simulink model "sampleModel364"  (R2021b)
settings: Solver=VariableStepAuto  StartTime=0.0  StopTime=10.0  RelTol=1e-3
undefined symbols (not defined in the file or in its folder): DiscIntNeverNeededParam, Newton, Raphson
libraries: simulink x11, slpidlib x2
settings Model: Creator=user  LastModifiedBy=user

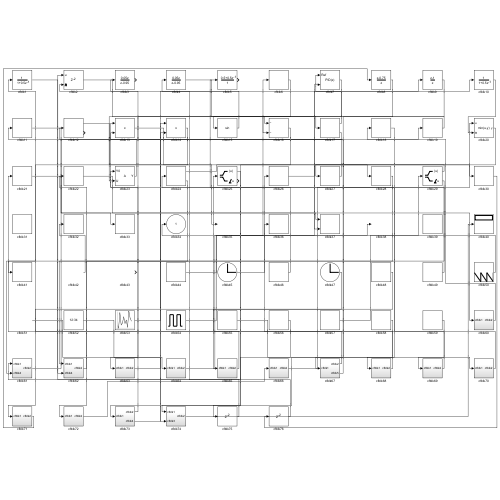
[thumbnail: Simulink's stored preview of the top-level diagram]
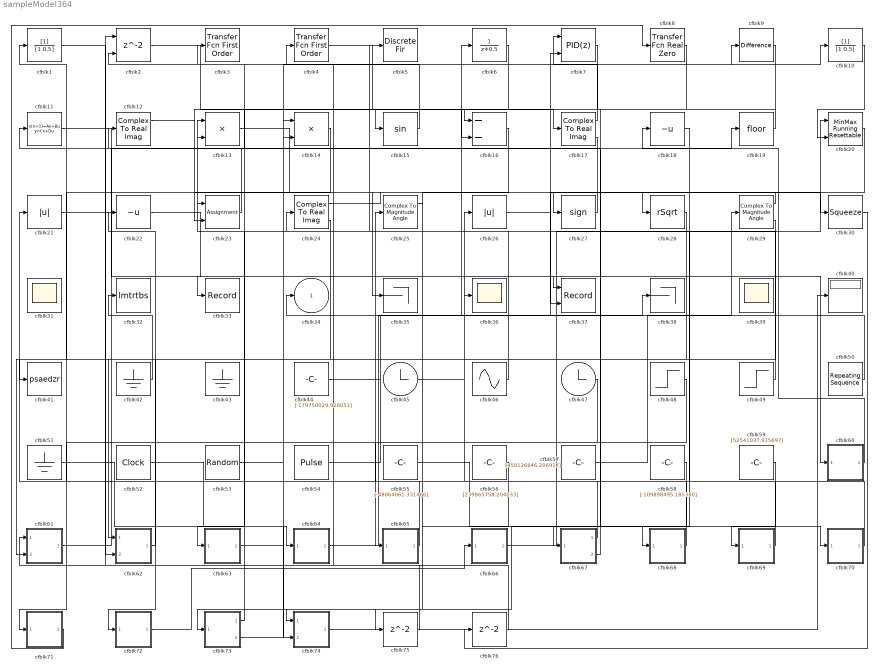
== system sampleModel364 ==
  cfblk1 : DiscreteFilter  SampleTime=1
  cfblk10 : DiscreteFilter  SampleTime=1
  cfblk11 : DiscreteStateSpace
  cfblk12 : ComplexToRealImag
  cfblk13 : Product
  cfblk14 : Product
  cfblk15 : Trigonometry
  cfblk16 : Sum  Inputs=--
  cfblk17 : ComplexToRealImag
  cfblk18 : UnaryMinus
  cfblk19 : Rounding
  cfblk2 : Delay  ShowEnablePort=on  SampleTime=1
      settings: InputPortMap=u0,e6
  cfblk20 : simulink/Math Operations/MinMax Running Resettable  Function=min  vinit=0.0
  cfblk21 : Abs
  cfblk22 : UnaryMinus
  cfblk23 : Assignment  DiagnosticForDimensions=Warning  IndexOptions=Index vector (dialog)  Indices=1  OutputSizes=1
  cfblk24 : ComplexToRealImag
  cfblk25 : ComplexToMagnitudeAngle
  cfblk26 : Abs
  cfblk27 : Signum
  cfblk28 : Sqrt  Operator=rSqrt  AlgorithmType=Newton-Raphson  SaturateOnIntegerOverflow=on
  cfblk29 : ComplexToMagnitudeAngle
  cfblk3 : simulink/Discrete/Transfer Fcn First Order  PoleZ=0.95  ICPrevOutput=0.0  DoSatur=off
  cfblk30 : Squeeze
  cfblk31 : Scope
      settings: Floating=on
  cfblk32 : ToWorkspace  VariableName=lmtrtbs  SaveFormat=Timeseries  SampleTime=-1
  cfblk33 : Record  FileSettingsInternal="{\"entries\":[{\"content\":{\"excelSettings\":{\"content\":{},\"type\":\"Streamout.ExcelSettings\"}},\"type\":\"Streamout.FileSettingStorage\",\"uuid\":\"efb9514b-eb39-49fb-8193-be4ff1269e7a\"}],\"packageUris\":[\"http://schema.mathworks.com/mf0/streamout_blocks/R2020a\"],\"version\":\"1.0\"}"  SignalsInternal="{\"entries\":[{\"content\":{\"signals\":[{\"content\":{\"blockPath\":[\"sampleModel364/cfblk33\"],\"channel\":[],\"dimensions\":[1],\"domain\":\"sampleModel364/cfblk33\",\"lineColor\":\"#0072bd\",\"plots\":[1],\"port\":1,\"sid\":[\"\"],\"signalID\":15049,\"signalName\":\"cfblk21\"},\"type\":\"RecordBlkView.Signal\",\"uuid\":\"19dc1517-5a93-4edc-820c-dcf5ac46ff94\"}]},\"type\":\"RecordBlkView.InputSignals\",\"uuid\":\"c811df6d-3595-4dee-9df3-0c2b135d4dd7\"}],\"packageUris\":[\"http://schema.mathworks.com/mf0/streamout_blocks/R2020a\"],\"version\":\"1.0\"}"  VisualizationBindings="{\"sparklinesplugin\":{\"info\":[{\"bindingParametersList\":[],\"subplotID\":1}]}}"
  cfblk35 : Terminator
  cfblk36 : Scope
  cfblk37 : Record  FileSettingsInternal="{\"entries\":[{\"content\":{\"excelSettings\":{\"content\":{},\"type\":\"Streamout.ExcelSettings\"}},\"type\":\"Streamout.FileSettingStorage\",\"uuid\":\"e2a7b882-2422-4f38-8975-ecb5b9b0d6a4\"}],\"packageUris\":[\"http://schema.mathworks.com/mf0/streamout_blocks/R2020a\"],\"version\":\"1.0\"}"  Layout=[1 1]  SignalsInternal="{\"entries\":[{\"content\":{\"signals\":[{\"content\":{\"blockPath\":[\"sampleModel364/cfblk37\"],\"channel\":[],\"dimensions\":[1],\"domain\":\"sampleModel364/cfblk37\",\"lineColor\":\"#a2142f\",\"plots\":[1],\"port\":1,\"sid\":[\"\"],\"signalID\":15041,\"signalName\":\"cfblk11\"},\"type\":\"RecordBlkView.Signal\",\"uuid\":\"8bbf27e7-d6ab-404e-982e-e11606491116\"},{\"content\":{\"blockPath\":[\"sampleModel364/cfblk37\"],\"channel\":[],\"dimensions\":[1],\"domain\":\"sampleModel364/cfblk37\",\"lineColor\":\"#139fff\",\"plots\":[1],\"port\":2,\"sid\":[\"\"],\"signalID\":15045,\"signalName\":\"cfblk20\"},\"type\":\"RecordBlkView.Signal\",\"uuid\":\"d022dd17-1fd8-4305-9f89-9d03c1f5384f\"}]},\"type\":\"RecordBlkView.InputSignals\",\"uuid\":\"b0c6aa1a-cfa3-4be9-9be2-43c7654ec479\"}],\"packageUris\":[\"http://schema.mathworks.com/mf0/streamout_blocks/R2020a\"],\"version\":\"1.0\"}"  VisualizationBindings="{\"xyplotplugin\":{\"info\":[{\"series\":[{\"bindingParametersList\":[{\"parameter\":\"X-Axis\",\"signalID\":15041,\"signalName\":\"cfblk11\"},{\"parameter\":\"Y-Axis\",\"signalID\":15045,\"signalName\":\"cfblk20\"}],\"seriesID\":3754}],\"subplotID\":1}]}}"  CompatibilityTag=XY
  cfblk38 : Terminator
  cfblk39 : Scope
      settings: Floating=on
  cfblk4 : simulink/Discrete/Transfer Fcn First Order  PoleZ=0.95  ICPrevOutput=0.0  DoSatur=off
  cfblk40 : Display
  cfblk41 : ToWorkspace  VariableName=psaedzr  SaveFormat=Timeseries  SampleTime=-1
  cfblk42 : Ground
  cfblk43 : Ground
  cfblk44 : Constant  Value=[-179750029.926051]  SampleTime=1
  cfblk45 : Clock
  cfblk46 : Sin  Amplitude=[258865866.152019]  Bias=[76546050.477614]  SampleTime=0
  cfblk47 : Clock
  cfblk48 : Step  Time=[28.000000]  Before=[914174276.713515]  After=[433065925.767623]  SampleTime=0
  cfblk49 : Step  Time=[16.000000]  Before=[-678100885.118563]  After=[625681601.472301]  SampleTime=0
  cfblk5 : DiscreteFir  SampleTime=1
  cfblk50 : simulink/Sources/Repeating Sequence  rep_seq_t=[0 2]  rep_seq_y=[-313407330.897961, -602777563.387411]
  cfblk51 : Ground
  cfblk52 : DigitalClock
  cfblk53 : UniformRandomNumber  Minimum=[-9430328336.158092]  Maximum=[6561492100.222932]  Seed=[48463456.000000]  SampleTime=0.1
  cfblk54 : DiscretePulseGenerator  PulseType=Time based  Amplitude=[255418173.633285]  Period=[59331713.081487]  PulseWidth=5  PhaseDelay=[5.000000]
  cfblk55 : Constant  Value=[-48864061.331466]  SampleTime=1
  cfblk56 : Constant  Value=[239865758.204033]  SampleTime=1
  cfblk57 : Constant  Value=[450126646.206917]  SampleTime=1
  cfblk58 : Constant  Value=[-109898495.185380]  SampleTime=1
  cfblk59 : Constant  Value=[52541037.915697]  SampleTime=1
  cfblk6 : DiscreteTransferFcn  SampleTime=1
  cfblk60 : Subsystem
  cfblk61 : Subsystem
  cfblk62 : Subsystem
  cfblk63 : Subsystem
  cfblk64 : Subsystem
  cfblk65 : Subsystem
  cfblk66 : Subsystem
  cfblk67 : Subsystem
  cfblk68 : Subsystem
  cfblk69 : Subsystem
  cfblk7 : slpidlib/PID Controller (2DOF)  Controller=PID  Form=Parallel  TimeDomain=Discrete-time  UseExternalTs=off  SampleTime=1  IntegratorMethod=Forward Euler  FilterMethod=Forward Euler  ControllerParametersSource=internal  P=1  I=1  D=0  UseFilter=on  N=100  b=1  c=1  TunerSelectOption=Transfer Function Based (PID Tuner App)  InitialConditionSource=internal  InitialConditionForIntegrator=0  InitialConditionForFilter=0  DifferentiatorICPrevScaledInput=0  ExternalReset=none  TrackingMode=off  Kt=1  LimitOutput=off  SatLimitsSource=internal  UpperSaturationLimit=inf  LowerSaturationLimit=-inf  LinearizeAsGain=off  AntiWindupMode=none  Kb=1  POutMin=[]  POutMax=[]  IOutMin=[]  IOutMax=[]  DOutMin=[]  DOutMax=[]  NOutMin=[]  NOutMax=[]  bOutMin=[]  bOutMax=[]  cOutMin=[]  cOutMax=[]  SumOutMin=[]  SumOutMax=[]  SaturationOutMin=[]  SaturationOutMax=[]  PParamMin=[]  PParamMax=[]  IParamMin=[]  IParamMax=[]  DParamMin=[]  DParamMax=[]  NParamMin=[]  NParamMax=[]  bParamMin=[]  bParamMax=[]  cParamMin=[]  cParamMax=[]  KbParamMin=[]  KbParamMax=[]  KtParamMin=[]  KtParamMax=[]  KbOutMin=[]  KbOutMax=[]  KtOutMin=[]  KtOutMax=[]  IntegratorOutMin=[]  IntegratorOutMax=[]  FilterOutMin=[]  FilterOutMax=[]  SumI1OutMin=[]  SumI1OutMax=[]  SumI2OutMin=[]  SumI2OutMax=[]  SumI3OutMin=[]  SumI3OutMax=[]  SumI4OutMin=[]  SumI4OutMax=[]  SumDOutMin=[]  SumDOutMax=[]  Sum1OutMin=[]  Sum1OutMax=[]  Sum2OutMin=[]  Sum2OutMax=[]  Sum3OutMin=[]  Sum3OutMax=[]  DifferentiatorOutMin=[]  DifferentiatorOutMax=[]  FilterDiffOutCoefMin=[]  FilterDiffOutCoefMax=[]  ReciprocalOutMin=[]  ReciprocalOutMax=[]  SumDenOutMin=[]  SumDenOutMax=[]  SumNumOutMin=[]  SumNumOutMax=[]  DivideOutMin=[]  DivideOutMax=[]  UdiffTsProdOutMin=[]  UdiffTsProdOutMax=[]  NTsProdOutMin=[]  NTsProdOutMax=[]  UintegralTsProdOutMin=[]  UintegralTsProdOutMax=[]  UngainTsProdOutMin=[]  UngainTsProdOutMax=[]  IntegratorContinuousStateAttributes=''  IntegratorStateMustResolveToSignalObject=off  IntegratorRTWStateStorageClass=Auto  FilterContinuousStateAttributes=''  FilterStateMustResolveToSignalObject=off  FilterRTWStateStorageClass=Auto  ParallelPVariant=InternalParameters  IdealPVariant=Disabled  IVariant=InternalParameters  DVariant=InternalParameters  bVariant=InternalParameters  cVariant=InternalParameters  IntegratorVariant=Discrete  SatVariant=Disabled  AWVariant=Passthrough  PCopyVariant=Disabled  TRVariant=Disabled  FdbkBlocksVariant=Forward  IdealPFdbkVariant=Disabled  SatFdbkVariant=Disabled  DerivativeFilterVariant=ForwardEulerFilter  NVariant=InternalParameters  NCopyVariant=Disabled  FilterICVariant=InternalICsFilter  IntegratorICVariant=InternalICs  ExternalResetVariant=Disabled  TRSumVariant=Passthrough  SumFdbkVariant=Disabled  SumVariant=Sum_PID  TsampFilterVariant=InternalTs  TsampNgainVariant=Passthrough  TsampIntegralVariant=Passthrough  ExternalSaturationOutDataTypeStr=Inherit: Same as second input
      settings: SourceProductBaseCode=SL
  cfblk70 : Subsystem
  cfblk71 : Subsystem
  cfblk72 : Subsystem
  cfblk73 : Subsystem
  cfblk74 : Subsystem
  cfblk75 : Delay  SampleTime=1
  cfblk76 : Delay  SampleTime=1
  cfblk8 : simulink/Discrete/Transfer Fcn Real Zero  ZeroZ=0.75  ICPrevInput=0.0  DoSatur=off
      settings: SourceProductBaseCode=SL
  cfblk9 : simulink/Discrete/Difference  ICPrevInput=0.0  OutMin=[]  OutMax=[]  OutDataTypeStr=Inherit: Inherit via back propagation  OutDataType=fixdt(1, 16)  OutScaling=2^-10  DoSatur=off
  cfblk34 : Outport
  wires:
  cfblk29/1 -> cfblk27/1
  cfblk64/1(cfblk2) -> cfblk38/1
  cfblk19/1 -> cfblk15/1
  cfblk60/1(cfblk2) -> cfblk18/1
  cfblk56/1 -> cfblk61/1(cfblk1)
  cfblk69/1(cfblk2) -> cfblk5/1
  cfblk58/1 -> cfblk73/1(cfblk1)
  cfblk28/1 -> cfblk61/2(cfblk4)
  cfblk65/1(cfblk2) -> cfblk21/1
  cfblk61/1(cfblk2) -> cfblk19/1
  cfblk49/1 -> cfblk13/1
  cfblk55/1 -> cfblk70/1(cfblk1)
  cfblk66/1(cfblk2) -> cfblk20/1
  cfblk47/1 -> cfblk71/1(cfblk1)
  cfblk45/1 -> cfblk26/1
  cfblk11/1 -> cfblk37/1
  cfblk53/1 -> cfblk14/1
  cfblk51/1 -> cfblk64/1(cfblk1)
  cfblk71/1(cfblk2) -> cfblk8/1
  cfblk20/1 -> cfblk37/2
  cfblk21/1 -> cfblk33/1
  cfblk29/2 -> cfblk62/1(cfblk1)
  cfblk17/1 -> cfblk7/1
  cfblk1/1 -> cfblk62/2(cfblk4)
  cfblk22/1 -> cfblk60/1(cfblk1)
  cfblk72/1(cfblk2) -> cfblk66/1(cfblk1)
  cfblk67/1(cfblk2) -> cfblk1/1
  cfblk42/1 -> cfblk32/1
  cfblk59/1 -> cfblk69/1(cfblk1)
  cfblk70/1(cfblk2) -> cfblk36/1
  cfblk50/1 -> cfblk34/1
  cfblk14/1 -> cfblk41/1
  cfblk68/1(cfblk2) -> cfblk25/1
  cfblk44/1 -> cfblk6/1
  cfblk24/1 -> cfblk30/1
  cfblk73/1(cfblk2) -> cfblk23/1
  cfblk25/1 -> cfblk74/1(cfblk1)
  cfblk62/1(cfblk2) -> cfblk22/1
  cfblk6/1 -> cfblk23/2
  cfblk2/1 -> cfblk16/1
  cfblk48/1 -> cfblk65/1(cfblk1)
  cfblk4/1 -> cfblk17/1
  cfblk10/1 -> cfblk20/2
  cfblk54/1 -> cfblk7/2
  cfblk26/1 -> cfblk9/1
  cfblk74/1(cfblk2) -> cfblk40/1
  cfblk9/1 -> cfblk67/1(cfblk1)
  cfblk18/1 -> cfblk68/1(cfblk1)
  cfblk17/2 -> cfblk11/1
  cfblk67/2(cfblk5) -> cfblk13/2
  cfblk13/1 -> cfblk35/1
  cfblk15/1 -> cfblk2/2
  cfblk24/2 -> cfblk72/1(cfblk1)
  cfblk12/1 -> cfblk28/1
  cfblk63/1(cfblk2) -> cfblk10/1
  cfblk23/1 -> cfblk12/1
  cfblk57/1 -> cfblk29/1
  cfblk27/1 -> cfblk3/1
  cfblk52/1 -> cfblk74/2(cfblk3)
  cfblk73/2(cfblk4) -> cfblk14/2
  cfblk8/1 -> cfblk16/2
  cfblk46/1 -> cfblk4/1
  cfblk7/1 -> cfblk63/1(cfblk1)
  cfblk16/1 -> cfblk75/1
  cfblk75/1 -> cfblk2/1
  cfblk30/1 -> cfblk76/1
  cfblk76/1 -> cfblk24/1

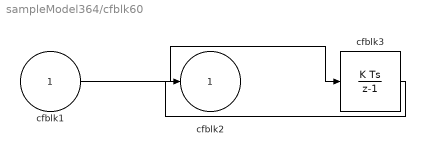
== system sampleModel364/cfblk60 ==
  cfblk1 : Inport
  cfblk3 : DiscreteIntegrator  ICPrevOutput=DiscIntNeverNeededParam  ICPrevScaledInput=DiscIntNeverNeededParam
  cfblk2 : Outport
  wires:
  cfblk1/1 -> cfblk3/1
  cfblk3/1 -> cfblk2/1

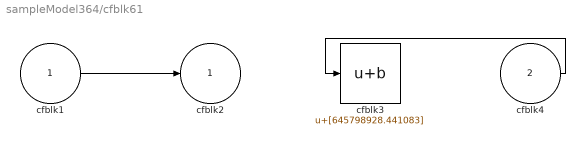
== system sampleModel364/cfblk61 ==
  cfblk1 : Inport
  cfblk4 : Inport  Port=2
  cfblk3 : Bias  Bias=[645798928.441083]
  cfblk2 : Outport
  wires:
  cfblk1/1 -> cfblk2/1
  cfblk4/1 -> cfblk3/1

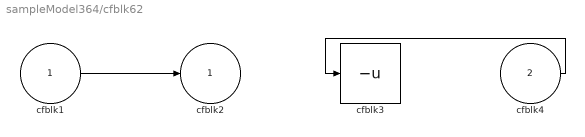
== system sampleModel364/cfblk62 ==
  cfblk1 : Inport
  cfblk4 : Inport  Port=2
  cfblk3 : UnaryMinus
  cfblk2 : Outport
  wires:
  cfblk4/1 -> cfblk3/1
  cfblk1/1 -> cfblk2/1

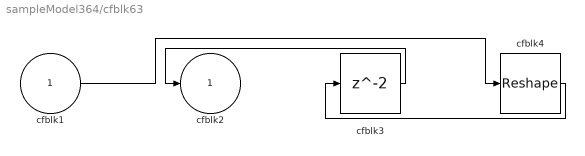
== system sampleModel364/cfblk63 ==
  cfblk1 : Inport
  cfblk3 : Delay  SampleTime=1
  cfblk4 : Reshape
  cfblk2 : Outport
  wires:
  cfblk3/1 -> cfblk2/1
  cfblk4/1 -> cfblk3/1
  cfblk1/1 -> cfblk4/1

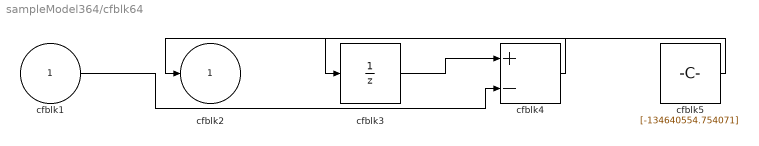
== system sampleModel364/cfblk64 ==
  cfblk1 : Inport
  cfblk3 : UnitDelay  HasFrameUpgradeWarning=on
  cfblk4 : Sum  Inputs=+-
  cfblk5 : Constant  Value=[-134640554.754071]  SampleTime=1
  cfblk2 : Outport
  wires:
  cfblk4/1 -> cfblk2/1
  cfblk3/1 -> cfblk4/1
  cfblk1/1 -> cfblk4/2
  cfblk5/1 -> cfblk3/1

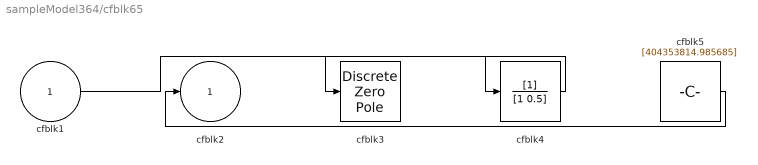
== system sampleModel364/cfblk65 ==
  cfblk1 : Inport
  cfblk3 : DiscreteZeroPole  Poles=[0 0.5]  Gain=1
  cfblk4 : DiscreteFilter  SampleTime=1
  cfblk5 : Constant  Value=[404353814.985685]  SampleTime=1
  cfblk2 : Outport
  wires:
  cfblk4/1 -> cfblk3/1
  cfblk5/1 -> cfblk2/1
  cfblk1/1 -> cfblk4/1

== system sampleModel364/cfblk66 ==
  cfblk1 : Inport
  cfblk3 : Signum
  cfblk2 : Outport
  wires:
  cfblk3/1 -> cfblk2/1
  cfblk1/1 -> cfblk3/1

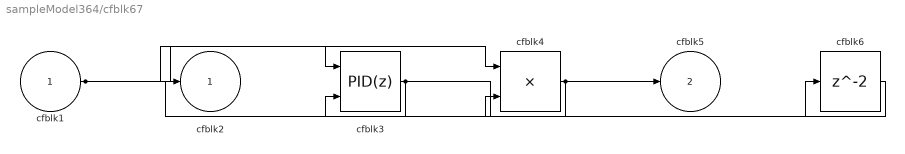
== system sampleModel364/cfblk67 ==
  cfblk1 : Inport
  cfblk3 : slpidlib/PID Controller (2DOF)  Controller=PID  Form=Parallel  TimeDomain=Discrete-time  UseExternalTs=off  SampleTime=1  IntegratorMethod=Forward Euler  FilterMethod=Forward Euler  ControllerParametersSource=internal  P=1  I=1  D=0  UseFilter=on  N=100  b=1  c=1  TunerSelectOption=Transfer Function Based (PID Tuner App)  InitialConditionSource=internal  InitialConditionForIntegrator=0  InitialConditionForFilter=0  DifferentiatorICPrevScaledInput=0  ExternalReset=none  TrackingMode=off  Kt=1  LimitOutput=off  SatLimitsSource=internal  UpperSaturationLimit=inf  LowerSaturationLimit=-inf  LinearizeAsGain=off  AntiWindupMode=none  Kb=1  POutMin=[]  POutMax=[]  IOutMin=[]  IOutMax=[]  DOutMin=[]  DOutMax=[]  NOutMin=[]  NOutMax=[]  bOutMin=[]  bOutMax=[]  cOutMin=[]  cOutMax=[]  SumOutMin=[]  SumOutMax=[]  SaturationOutMin=[]  SaturationOutMax=[]  PParamMin=[]  PParamMax=[]  IParamMin=[]  IParamMax=[]  DParamMin=[]  DParamMax=[]  NParamMin=[]  NParamMax=[]  bParamMin=[]  bParamMax=[]  cParamMin=[]  cParamMax=[]  KbParamMin=[]  KbParamMax=[]  KtParamMin=[]  KtParamMax=[]  KbOutMin=[]  KbOutMax=[]  KtOutMin=[]  KtOutMax=[]  IntegratorOutMin=[]  IntegratorOutMax=[]  FilterOutMin=[]  FilterOutMax=[]  SumI1OutMin=[]  SumI1OutMax=[]  SumI2OutMin=[]  SumI2OutMax=[]  SumI3OutMin=[]  SumI3OutMax=[]  SumI4OutMin=[]  SumI4OutMax=[]  SumDOutMin=[]  SumDOutMax=[]  Sum1OutMin=[]  Sum1OutMax=[]  Sum2OutMin=[]  Sum2OutMax=[]  Sum3OutMin=[]  Sum3OutMax=[]  DifferentiatorOutMin=[]  DifferentiatorOutMax=[]  FilterDiffOutCoefMin=[]  FilterDiffOutCoefMax=[]  ReciprocalOutMin=[]  ReciprocalOutMax=[]  SumDenOutMin=[]  SumDenOutMax=[]  SumNumOutMin=[]  SumNumOutMax=[]  DivideOutMin=[]  DivideOutMax=[]  UdiffTsProdOutMin=[]  UdiffTsProdOutMax=[]  NTsProdOutMin=[]  NTsProdOutMax=[]  UintegralTsProdOutMin=[]  UintegralTsProdOutMax=[]  UngainTsProdOutMin=[]  UngainTsProdOutMax=[]  IntegratorContinuousStateAttributes=''  IntegratorStateMustResolveToSignalObject=off  IntegratorRTWStateStorageClass=Auto  FilterContinuousStateAttributes=''  FilterStateMustResolveToSignalObject=off  FilterRTWStateStorageClass=Auto  ParallelPVariant=InternalParameters  IdealPVariant=Disabled  IVariant=InternalParameters  DVariant=InternalParameters  bVariant=InternalParameters  cVariant=InternalParameters  IntegratorVariant=Discrete  SatVariant=Disabled  AWVariant=Passthrough  PCopyVariant=Disabled  TRVariant=Disabled  FdbkBlocksVariant=Forward  IdealPFdbkVariant=Disabled  SatFdbkVariant=Disabled  DerivativeFilterVariant=ForwardEulerFilter  NVariant=InternalParameters  NCopyVariant=Disabled  FilterICVariant=InternalICsFilter  IntegratorICVariant=InternalICs  ExternalResetVariant=Disabled  TRSumVariant=Passthrough  SumFdbkVariant=Disabled  SumVariant=Sum_PID  TsampFilterVariant=InternalTs  TsampNgainVariant=Passthrough  TsampIntegralVariant=Passthrough  ExternalSaturationOutDataTypeStr=Inherit: Same as second input
      settings: SourceProductBaseCode=SL
  cfblk4 : Product
  cfblk6 : Delay  SampleTime=1
  cfblk2 : Outport
  cfblk5 : Outport  Port=2
  wires:
  cfblk1/1 -> cfblk4/1, cfblk3/1
  cfblk3/1 -> cfblk2/1, cfblk6/1
  cfblk4/1 -> cfblk5/1, cfblk3/2
  cfblk6/1 -> cfblk4/2

== system sampleModel364/cfblk68 ==
  cfblk1 : Inport
  cfblk3 : DiscreteFilter  SampleTime=1
  cfblk2 : Outport
  wires:
  cfblk3/1 -> cfblk2/1
  cfblk1/1 -> cfblk3/1

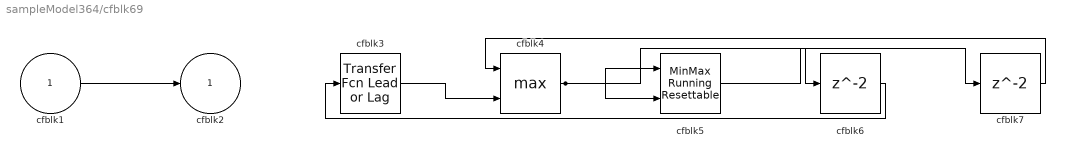
== system sampleModel364/cfblk69 ==
  cfblk1 : Inport
  cfblk3 : simulink/Discrete/Transfer Fcn Lead or Lag  PoleZ=0.95  ZeroZ=0.75  ICPrevOutput=0.0  ICPrevInput=0.0  DoSatur=off
      settings: SourceProductBaseCode=SL
  cfblk4 : MinMax  Function=max  Inputs=2
  cfblk5 : simulink/Math Operations/MinMax Running Resettable  Function=min  vinit=0.0
  cfblk6 : Delay  SampleTime=1
  cfblk7 : Delay  SampleTime=1
  cfblk2 : Outport
  wires:
  cfblk1/1 -> cfblk2/1
  cfblk3/1 -> cfblk4/2
  cfblk4/1 -> cfblk5/1, cfblk5/2, cfblk6/1
  cfblk6/1 -> cfblk3/1
  cfblk5/1 -> cfblk7/1
  cfblk7/1 -> cfblk4/1

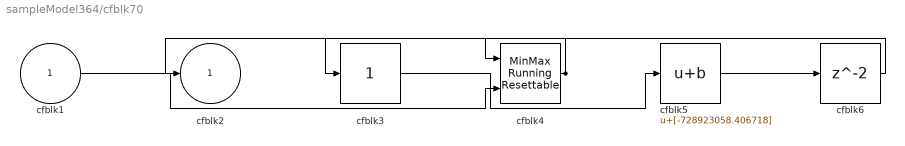
== system sampleModel364/cfblk70 ==
  cfblk1 : Inport
  cfblk3 : simulink/Math Operations/Slider Gain  gain=1  low=0  high=2
  cfblk4 : simulink/Math Operations/MinMax Running Resettable  Function=min  vinit=0.0
  cfblk5 : Bias  Bias=[-728923058.406718]
  cfblk6 : Delay  SampleTime=1
  cfblk2 : Outport
  wires:
  cfblk3/1 -> cfblk5/1
  cfblk1/1 -> cfblk4/2
  cfblk4/1 -> cfblk3/1, cfblk2/1
  cfblk5/1 -> cfblk6/1
  cfblk6/1 -> cfblk4/1

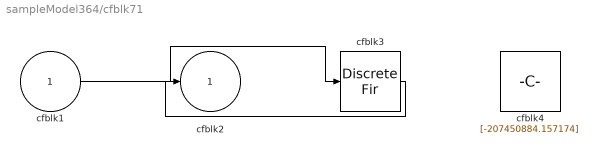
== system sampleModel364/cfblk71 ==
  cfblk1 : Inport
  cfblk3 : DiscreteFir  SampleTime=1
  cfblk4 : Constant  Value=[-207450884.157174]  SampleTime=1
  cfblk2 : Outport
  wires:
  cfblk1/1 -> cfblk3/1
  cfblk3/1 -> cfblk2/1

== system sampleModel364/cfblk72 ==
  cfblk1 : Inport
  cfblk3 : simulink/Discrete/Transfer Fcn First Order  PoleZ=0.95  ICPrevOutput=0.0  DoSatur=off
  cfblk2 : Outport
  wires:
  cfblk1/1 -> cfblk3/1
  cfblk3/1 -> cfblk2/1

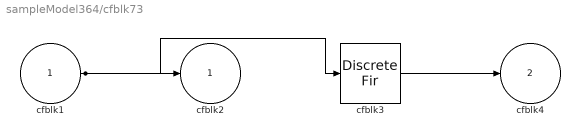
== system sampleModel364/cfblk73 ==
  cfblk1 : Inport
  cfblk3 : DiscreteFir  SampleTime=1
  cfblk2 : Outport
  cfblk4 : Outport  Port=2
  wires:
  cfblk1/1 -> cfblk2/1, cfblk3/1
  cfblk3/1 -> cfblk4/1

== system sampleModel364/cfblk74 ==
  cfblk1 : Inport
  cfblk3 : Inport  Port=2
  cfblk2 : Outport
  wires:
  cfblk3/1 -> cfblk2/1
